simulink model "B4_quadcopter_model_discrete"  (R2021b)
settings: Solver=VariableStepAuto  StartTime=0.0  StopTime=10  FixedStep=0.002  RelTol=1e-3
values from neighbouring files (symbols this model uses):
  coef_sim_1 = tf_des_d.Denominator{1}(2)    [A11_setup_script_pprz.m]    (also in A1_setup_script.m; A6_slow_actuator.m)
  coef_sim_2 = tf_des_d.Numerator{1}(2)    [A11_setup_script_pprz.m]    (also in A1_setup_script.m; A6_slow_actuator.m)
  doublet_mag = - 0.15    (= -0.15)    [A11_setup_script_pprz.m]    (also in A1_setup_script.m)
  doublet_time = 6    [A11_setup_script_pprz.m]    (also in A1_setup_script.m)
  f_8 = 1    [A11_setup_script_pprz.m]    (also in A1_setup_script.m)
  FILT_CUTOFF = 2*pi*5    (= 31.4159265359)    [A11_setup_script_pprz.m]    (also in A1_setup_script.m)
  FILTER = 1    [A11_setup_script_pprz.m]    (also in A1_setup_script.m)
  G1 = inv(I)*G1_r    [A10_simple_plant.m]    (also in A11_setup_script_pprz.m = G1/scale; A1_setup_script.m = [G1;G1_T])
  G1_simple = inv(I)*G1_r_simple    [A1_setup_script.m]
  G2 = G2/scale    [A11_setup_script_pprz.m]    (also in A1_setup_script.m = (1/sampling_time)*inv(I)*(G2_r))
  h_plate = 0.3    [A11_setup_script_pprz.m]    (also in A1_setup_script.m = 0.16)
  I = eye(3,3)    [A10_simple_plant.m]    (also in A11_setup_script_pprz.m; A1_setup_script.m; A2_B_matrix_generation_symbolic.m = [Ixx 0 0; A3_B_matrix_generation_symbolic_cascaded.m = [Ixx 0 0)
  Iyy = 0.0008    [A11_setup_script_pprz.m]    (also in A1_setup_script.m = 0.0015)
  Izz = 0.000498    [A11_setup_script_pprz.m]    (also in A1_setup_script.m = 0.00015)
  K = 7    [A11_setup_script_pprz.m]    (also in A1_setup_script.m = 10)
  K_act = 50    [A10_simple_plant.m]    (also in A11_setup_script_pprz.m = 20; A1_setup_script.m = 20)
  K_act_outer = diag([K K K_act])    [A1_setup_script.m]
  K_d = 15    [A11_setup_script_pprz.m]    (also in A1_setup_script.m = 25)
  K_dd = K_act    (= 20)    [A11_setup_script_pprz.m]    (also in A1_setup_script.m)
  K_dyn = K    (= 10)    [A1_setup_script.m]
  K_ec = 50    [A11_setup_script_pprz.m]    (also in A1_setup_script.m = 251)
  K_ec_d = 13    [A11_setup_script_pprz.m]    (also in A1_setup_script.m = 25)
  K_ec_d_u = 1.5    [A11_setup_script_pprz.m]    (also in A1_setup_script.m = 5)
  K_ec_d_v = 1.5    [A11_setup_script_pprz.m]    (also in A1_setup_script.m = 5)
  K_ec_d_w = 1.5    [A11_setup_script_pprz.m]    (also in A1_setup_script.m = 5)
  K_ec_dd = 9    [A11_setup_script_pprz.m]    (also in A1_setup_script.m = 45)
  K_ec_i = 0    [A11_setup_script_pprz.m]    (also in A1_setup_script.m = 380)
  K_ec_u = 1.5    [A11_setup_script_pprz.m]    (also in A1_setup_script.m = 5)
  K_ec_v = 1.5    [A11_setup_script_pprz.m]    (also in A1_setup_script.m = 5)
  K_ec_w = 1.5    [A11_setup_script_pprz.m]    (also in A1_setup_script.m = 5)
  K_t = 0.0005    [A10_simple_plant.m]    (also in A11_setup_script_pprz.m = 6.557e-08; A1_setup_script.m = 6.557e-08)
  K_u = 1.0    (= 1)    [A11_setup_script_pprz.m]    (also in A1_setup_script.m = 1.5)
  K_u_d = 2.5    [A11_setup_script_pprz.m]    (also in A1_setup_script.m = 7)
  K_u_dd = K    (= 10)    [A1_setup_script.m]
  K_v = 1.0    (= 1)    [A11_setup_script_pprz.m]    (also in A1_setup_script.m = 1.5)
  K_v_d = 2.5    [A11_setup_script_pprz.m]    (also in A1_setup_script.m = 7)
  K_v_dd = K    (= 10)    [A1_setup_script.m]
  K_w = 1.0    (= 1)    [A11_setup_script_pprz.m]    (also in A1_setup_script.m = 4.5)
  K_w_d = 2.5    [A11_setup_script_pprz.m]    (also in A1_setup_script.m = 7)
  K_w_dd = K    (= 10)    [A1_setup_script.m]
  l_plate = 0.1    [A11_setup_script_pprz.m]    (also in A1_setup_script.m = 0.11)
  m = 0.4    [A10_simple_plant.m]    (also in A11_setup_script_pprz.m; A1_setup_script.m)
  NOISE = 0    [A11_setup_script_pprz.m]    (also in A1_setup_script.m)
  NOISE_ACC = 0.00005    (= 5e-05)    [A11_setup_script_pprz.m]    (also in A1_setup_script.m)
  NOISE_GYRO = 0.00005    (= 5e-05)    [A11_setup_script_pprz.m]    (also in A1_setup_script.m)
  NOISE_RPM = 200    [A11_setup_script_pprz.m]    (also in A1_setup_script.m)
  omega_act = 50    [A6_slow_actuator.m]
  omega_des = 20.00    (= 20)    [A11_setup_script_pprz.m]    (also in A1_setup_script.m; A6_slow_actuator.m = 49)
  sampling_time = 1/frequency    (= 0.002)    [A11_setup_script_pprz.m]    (also in A12_sim_multi_run.m; A1_setup_script.m; A6_slow_actuator.m)
  scale_8 = 1.6    [A11_setup_script_pprz.m]    (also in A1_setup_script.m)
  start_8 = 2    [A11_setup_script_pprz.m]    (also in A1_setup_script.m)
  start_time = 2    [A11_setup_script_pprz.m]    (also in A1_setup_script.m = 1)
  t_8 = 10    [A11_setup_script_pprz.m]    (also in A1_setup_script.m)
  w_plate = 0.3    [A11_setup_script_pprz.m]    (also in A1_setup_script.m = 0.36)
undefined symbols (not defined in the file or in its folder): DiscIntNeverNeededParam, K_ec_d_p, K_ec_d_q, K_ec_d_r, K_ec_dd_p, K_ec_dd_q, K_ec_dd_r, K_ec_i_u, K_ec_i_v, K_ec_i_w, K_ec_p, K_ec_q, K_ec_r, K_p, K_p_d, K_p_dd, K_q, K_q_d, K_q_dd, K_r, K_r_d, K_r_dd
libraries: simulink x44, cstblocks x37, dspinverses x26, dspmathops x9, dspstat3 x9, aerolibutil x9, sharedutil x3, aerolibanim x1
(part 12 of 13)

== matlab function B4_quadcopter_model_discrete/Discrete Model/Discrete INDI Controller Cascaded w// Actuator Compensation/8-shape trajectory/MATLAB Function ==
  data: x output; t input; y output; f input; scale input; psi output; sampling_time input; total_time input; start_time input
function [x,y,psi] = inf_trajectory(t,f,scale,sampling_time,total_time,start_time)

t_norm = t/total_time;

x = 2*scale*sin(2*pi*f*t_norm);
y = scale*sin(2*pi*f*t_norm*2);

x_n = 2*scale*sin(2*pi*f*(t_norm+sampling_time));
y_n = scale*sin(2*pi*f*(t_norm+sampling_time)*2);

dx = x_n - x;
dy = y_n - y;

psi = atan2(dy,dx);

== matlab function B4_quadcopter_model_discrete/Discrete Model - Complementary Filtering/Discrete INDI Controller Cascaded w// Actuator Compensation/8-shape trajectory/MATLAB Function ==
  data: x output; t input; y output; f input; scale input; psi output; sampling_time input; total_time input; start_time input
function [x,y,psi] = inf_trajectory(t,f,scale,sampling_time,total_time,start_time)

t_norm = t/total_time;

x = 2*scale*sin(2*pi*f*t_norm);
y = scale*sin(2*pi*f*t_norm*2);

x_n = 2*scale*sin(2*pi*f*(t_norm+sampling_time));
y_n = scale*sin(2*pi*f*(t_norm+sampling_time)*2);

dx = x_n - x;
dy = y_n - y;

psi = atan2(dy,dx);

== matlab function B4_quadcopter_model_discrete/Discrete Model - Complementary Filtering/Discrete INDI Controller Cascaded w// Actuator Compensation/ERROR CONTROLLER ATTITUDE/MATLAB Function1 ==
  data: pis_e input; psie_w output
function psie_w = wrapper(pis_e)

if pis_e > pi
    psie_w = pis_e - 2*pi;
elseif pis_e <= -pi
    psie_w = pis_e + 2*pi;
else
    psie_w = pis_e;
end

== matlab function B4_quadcopter_model_discrete/Discrete Model/Discrete INDI Controller Cascaded w// Actuator Compensation Double/Pitch Jerk Compensation1/MATLAB Function ==
  data: Ax input; dtheta input; Vx input; theta input; Jx_comp output; w_plate input; h_plate input; m input
function Jx_comp = jerk_compensator(Ax,dtheta,Vx,theta,w_plate,h_plate,m)

S_plate = w_plate * h_plate;
rho = 1.225;
Vx_sign = sign(Vx);

Jx_comp = - (297*S_plate*Vx^2*Vx_sign*dtheta*rho)/(1000*m*pi) - (Ax*S_plate*Vx*Vx_sign*rho*((297*theta)/(500*pi) + 997/1000))/m;

== matlab function B4_quadcopter_model_discrete/Discrete Model/Discrete INDI Controller Cascaded w// Actuator Compensation Double/8-shape trajectory/MATLAB Function ==
  data: x output; t input; y output; f input; scale input; psi output; sampling_time input; total_time input; start_time input
function [x,y,psi] = inf_trajectory(t,f,scale,sampling_time,total_time,start_time)

t_norm = t/total_time;

x = 2*scale*sin(2*pi*f*t_norm);
y = scale*sin(2*pi*f*t_norm*2);

x_n = 2*scale*sin(2*pi*f*(t_norm+sampling_time));
y_n = scale*sin(2*pi*f*(t_norm+sampling_time)*2);

dx = x_n - x;
dy = y_n - y;

psi = atan2(dy,dx);

if psi > 2
    psi = psi - 2*pi;
end

== matlab function B4_quadcopter_model_discrete/Discrete Model/Discrete INDI Controller Cascaded w// Actuator Compensation Double/Drag Plate Aerodynamics/drag plate My ==
  data: w_plate input; h_plate input; l_plate input; theta input; Vx input; My_dp output; Fx_earth output; Fz_earth output; Cl output; Cd output
function [My_dp, Fx_earth, Fz_earth, Cl, Cd]= drag_plate_My(w_plate,h_plate,l_plate,theta,Vx)

% define constants
rho = 1.225;
S_plate = w_plate*h_plate;

% Drag Coefficient
Cd = 0.0033*(90+rad2deg(theta))+0.7;

% Lift Coefficient
Cl = -0.0228*(90+rad2deg(theta))+2.01;

% get drag and lift
D_plate = 0.5*rho*Vx^2*S_plate*Cd;
L_plate = 0.5*rho*Vx^2*S_plate*Cl;
R_plate = sqrt(D_plate^2 + L_plate^2);

% get the moment caused by the drag
My_dp = l_plate*R_plate;

% get the forces caused by the drag
Fx_earth = -D_plate*sign(Vx);
Fz_earth = -L_plate;

== matlab function B4_quadcopter_model_discrete/Discrete Model/Discrete INDI Controller Cascaded w// Actuator Compensation/body rates to euler rates/pqr_to_euler_rates ==
  data: Phi input; T output; Theta input
function T = pqr_to_euler_rates(Phi,Theta)
T = [1 (sin(Phi)*sin(Theta))/cos(Theta) (cos(Phi)*sin(Theta))/cos(Theta);
0 cos(Phi) -sin(Phi);
0 sin(Phi)/cos(Theta) cos(Phi)/cos(Theta)];

== matlab function B4_quadcopter_model_discrete/Discrete Model/Discrete INDI Controller Cascaded w// Actuator Compensation Double/G1+G2 ==
  data: G1 input; B_inner output; G2 input; omega input; K_act input
function B_inner = B_inner(G1,G2,omega,K_act)

% add additional row to G2 for equal size
G2_T = [0 0 0 0];
G2 = vertcat(G2,G2_T);

B_inner = K_act*(G1 .* omega' + G2);

== matlab function B4_quadcopter_model_discrete/Discrete Model/Discrete INDI Controller Cascaded w// Actuator Compensation Double/G2_comp ==
  data: G2 input; K_act input; domega input; G2_comp output
function G2_comp = G2_comp(G2,K_act,domega)

G2_comp = K_act * G2(3,:) * domega;

== matlab function B4_quadcopter_model_discrete/Discrete Model/Discrete INDI Controller Cascaded w// Actuator Compensation Double/MATLAB Function1 ==
  data: T input; B_outer output; Phi input; Theta input; Psi input; m input; K_act_outer input
function B_outer = control_allocation_simple_outer(T,Phi,Theta,Psi,m,K_act_outer)

B_outer = zeros(3,3);

B_outer(1,1) = (T*cos(Phi)*cos(Psi)*cos(Theta))/m;
B_outer(2,1) = (T*cos(Phi)*cos(Theta)*sin(Psi))/m;
B_outer(3,1) = -(T*cos(Phi)*sin(Theta))/m;

B_outer(1,2) = (T*(cos(Phi)*sin(Psi) - cos(Psi)*sin(Phi)*sin(Theta)))/m;
B_outer(2,2) = -(T*(cos(Phi)*cos(Psi) + sin(Phi)*sin(Psi)*sin(Theta)))/m;
B_outer(3,2) = -(T*cos(Theta)*sin(Phi))/m;

B_outer(1,3) = (sin(Phi)*sin(Psi) + cos(Phi)*cos(Psi)*sin(Theta))/m;
B_outer(2,3) = -(cos(Psi)*sin(Phi) - cos(Phi)*sin(Psi)*sin(Theta))/m;
B_outer(3,3) = (cos(Phi)*cos(Theta))/m;

% compensate for actuator dynamics
B_outer = K_act_outer * B_outer;

end

== matlab function B4_quadcopter_model_discrete/Discrete Model/Discrete INDI Controller Cascaded w// Actuator Compensation Double/Pitch Jerk Compensation/MATLAB Function ==
  data: dx input; dy input; dz input; Phi input; Theta input; Psi input; ddx input; ddy input; ddz input; dPhi input; dTheta input; dPsi input; qdd_comp output; w_plate input; h_plate input; l_plate input; Iyy input
function qdd_comp = pitch_compensator(dx,dy,dz,Phi,Theta,Psi,ddx,ddy,ddz,dPhi,dTheta,dPsi,w_plate,h_plate,l_plate,Iyy)

% define constants
rho = 1.225;
S_plate = w_plate*h_plate;
Cd = 1.2;
Cl = 0.2;

% Q term
Q = (l_plate*rho*S_plate)/(Iyy*2);

% derivative vector
der_vect = [ddx ddy ddz dPhi dTheta dPsi];

% State terms
Fs_theta_dx = -Q*(Cd*cos(Theta) - Cl*sin(Theta))*(2*(sin(Phi)*sin(Psi) + cos(Phi)*cos(Psi)*sin(Theta))*(dx*(sin(Phi)*sin(Psi) + cos(Phi)*cos(Psi)*sin(Theta)) - dy*(cos(Psi)*sin(Phi) - cos(Phi)*sin(Psi)*sin(Theta)) + dz*cos(Phi)*cos(Theta)) + 2*cos(Psi)*cos(Theta)*(dx*cos(Psi)*cos(Theta) - dz*sin(Theta) + dy*cos(Theta)*sin(Psi)));
Fs_theta_dy = Q*(Cd*cos(Theta) - Cl*sin(Theta))*(2*(cos(Psi)*sin(Phi) - cos(Phi)*sin(Psi)*sin(Theta))*(dx*(sin(Phi)*sin(Psi) + cos(Phi)*cos(Psi)*sin(Theta)) - dy*(cos(Psi)*sin(Phi) - cos(Phi)*sin(Psi)*sin(Theta)) + dz*cos(Phi)*cos(Theta)) - 2*cos(Theta)*sin(Psi)*(dx*cos(Psi)*cos(Theta) - dz*sin(Theta) + dy*cos(Theta)*sin(Psi)));
Fs_theta_dz = Q*(Cd*cos(Theta) - Cl*sin(Theta))*(2*sin(Theta)*(dx*cos(Psi)*cos(Theta) - dz*sin(Theta) + dy*cos(Theta)*sin(Psi)) - 2*cos(Phi)*cos(Theta)*(dx*(sin(Phi)*sin(Psi) + cos(Phi)*cos(Psi)*sin(Theta)) - dy*(cos(Psi)*sin(Phi) - cos(Phi)*sin(Psi)*sin(Theta)) + dz*cos(Phi)*cos(Theta)));
Fs_theta_phi = 2*Q*(Cd*cos(Theta) - Cl*sin(Theta))*(dx*(sin(Phi)*sin(Psi) + cos(Phi)*cos(Psi)*sin(Theta)) - dy*(cos(Psi)*sin(Phi) - cos(Phi)*sin(Psi)*sin(Theta)) + dz*cos(Phi)*cos(Theta))*(dy*(cos(Phi)*cos(Psi) + sin(Phi)*sin(Psi)*sin(Theta)) - dx*(cos(Phi)*sin(Psi) - cos(Psi)*sin(Phi)*sin(Theta)) + dz*cos(Theta)*sin(Phi));
Fs_theta_theta = Q*(Cl*cos(Theta) + Cd*sin(Theta))*((dx*(sin(Phi)*sin(Psi) + cos(Phi)*cos(Psi)*sin(Theta)) - dy*(cos(Psi)*sin(Phi) - cos(Phi)*sin(Psi)*sin(Theta)) + dz*cos(Phi)*cos(Theta))^2 + (dx*cos(Psi)*cos(Theta) - dz*sin(Theta) + dy*cos(Theta)*sin(Psi))^2) + Q*(2*(dx*cos(Psi)*cos(Theta) - dz*sin(Theta) + dy*cos(Theta)*sin(Psi))*(dz*cos(Theta) + dx*cos(Psi)*sin(Theta) + dy*sin(Psi)*sin(Theta)) - 2*(dx*cos(Phi)*cos(Psi)*cos(Theta) - dz*cos(Phi)*sin(Theta) + dy*cos(Phi)*cos(Theta)*sin(Psi))*(dx*(sin(Phi)*sin(Psi) + cos(Phi)*cos(Psi)*sin(Theta)) - dy*(cos(Psi)*sin(Phi) - cos(Phi)*sin(Psi)*sin(Theta)) + dz*cos(Phi)*cos(Theta)))*(Cd*cos(Theta) - Cl*sin(Theta));
Fs_theta_psi = -Q*(Cd*cos(Theta) - Cl*sin(Theta))*(2*(dy*cos(Psi)*cos(Theta) - dx*cos(Theta)*sin(Psi))*(dx*cos(Psi)*cos(Theta) - dz*sin(Theta) + dy*cos(Theta)*sin(Psi)) + 2*(dx*(cos(Psi)*sin(Phi) - cos(Phi)*sin(Psi)*sin(Theta)) + dy*(sin(Phi)*sin(Psi) + cos(Phi)*cos(Psi)*sin(Theta)))*(dx*(sin(Phi)*sin(Psi) + cos(Phi)*cos(Psi)*sin(Theta)) - dy*(cos(Psi)*sin(Phi) - cos(Phi)*sin(Psi)*sin(Theta)) + dz*cos(Phi)*cos(Theta)));

Fs_theta_der = [Fs_theta_dx Fs_theta_dy Fs_theta_dz Fs_theta_phi Fs_theta_theta Fs_theta_psi];

% compensation term
qdd_comp = Fs_theta_der * der_vect';

== matlab function B4_quadcopter_model_discrete/Discrete Model/Discrete INDI Controller Cascaded w// Actuator Compensation Double/Pitch Jerk Compensation CopyPaste/Aero Package Easy/drag plate My ==
  data: w_plate input; h_plate input; l_plate input; theta input; u input; w input; My_dp output; Fx_earth output; Fz_earth output; Cl output; Cd output
function [My_dp, Fx_earth, Fz_earth, Cl, Cd]= drag_plate_My(w_plate,h_plate,l_plate,theta,u,w)

% define constants
rho = 1.225;
S_plate = w_plate*h_plate;

% Velocity vector
V = sqrt(u^2+w^2);

% % Drag Coefficient
% Cd = 0.0033*(90+rad2deg(theta))+0.7;
% 
% % Lift Coefficient
% Cl = -0.0228*(90+rad2deg(theta))+2.01;

Cd = 1.2;
Cl = 0.2;

% get drag and lift
D_plate = 0.5*rho*V^2*S_plate*Cd*sign(u);
L_plate = 0.5*rho*V^2*S_plate*Cl;

% get forces in body frame
Fx_body = - D_plate * cos(theta) + L_plate * sin(theta);
Fz_body = - D_plate * sin(theta) - L_plate * cos(theta);

% get the moment caused by the drag
My_dp = l_plate*Fx_body;

% get the forces caused by the drag
Fx_earth = - D_plate;
Fz_earth = L_plate;

== matlab function B4_quadcopter_model_discrete/Tester Block/Wrapping Test/MATLAB Function ==
  data: x output; t input; y output; f input; scale input; psi output; sampling_time input; total_time input; start_time input
function [x,y,psi] = inf_trajectory(t,f,scale,sampling_time,total_time,start_time)

t_norm = t/total_time;

x = 2*scale*sin(2*pi*f*t_norm);
y = scale*sin(2*pi*f*t_norm*2);

x_n = 2*scale*sin(2*pi*f*(t_norm+sampling_time));
y_n = scale*sin(2*pi*f*(t_norm+sampling_time)*2);

dx = x_n - x;
dy = y_n - y;

psi = atan2(dy,dx);

== matlab function B4_quadcopter_model_discrete/Discrete Model/Discrete INDI Controller Cascaded/G1+G2 ==
  data: G1 input; B_inner output; G2 input; omega input
function B_inner = B_inner(G1,G2,omega)

% add additional row to G2 for equal size
G2_T = [0 0 0 0];
G2 = vertcat(G2,G2_T);

B_inner = (G1 .* omega' + G2);

== matlab function B4_quadcopter_model_discrete/Tester Block/Wrapping Test/MATLAB Function1 ==
  data: pis_e input; psie_w output
function psie_w = wrapper(pis_e)

if pis_e > pi
    psie_w = pis_e - 2*pi;
elseif pis_e <= -pi
    psie_w = pis_e + 2*pi;
else
    psie_w = pis_e;
end

== matlab function B4_quadcopter_model_discrete/Tester Block/Wrapping Test/MATLAB Function2 ==
  data: psi_e_w input; psi_e output
function psi_e = unwrap(psi_e_w)

if psi_e_w > pi
    psi_e = psi_e_w - 2*pi;
elseif psi_e_w <= -pi
    psi_e = psi_e_w + 2*pi;
else
    psi_e = psi_e_w;
end

== matlab function B4_quadcopter_model_discrete/Discrete Model/Discrete INDI Controller Cascaded w// Actuator Compensation/INTERNAL REFERENCE MODEL ATTITUDE/MATLAB Function1 ==
  data: pis_e input; psie_w output
function psie_w = wrapper(pis_e)

if pis_e > pi
    psie_w = pis_e - 2*pi;
elseif pis_e <= -pi
    psie_w = pis_e + 2*pi;
else
    psie_w = pis_e;
end

== matlab function B4_quadcopter_model_discrete/Discrete Model/Plant and State Estimation/euler_rates_to_pqr ==
  data: Phi input; R output; Theta input
function R = euler_rates_to_pqr(Phi,Theta)
R = [1 0 -sin(Theta);
0 cos(Phi) cos(Theta)*sin(Phi);
0 -sin(Phi) cos(Phi)*cos(Theta)];

== matlab function B4_quadcopter_model_discrete/Discrete Model/Plant and State Estimation/pqr_to_euler_rates ==
  data: Phi input; T output; Theta input
function T = pqr_to_euler_rates(Phi,Theta)
T = [1 (sin(Phi)*sin(Theta))/cos(Theta) (cos(Phi)*sin(Theta))/cos(Theta);
0 cos(Phi) -sin(Phi);
0 sin(Phi)/cos(Theta) cos(Phi)/cos(Theta)];

== matlab function B4_quadcopter_model_discrete/Discrete Model/Discrete INDI Controller Cascaded/MATLAB Function1 ==
  data: T input; B_outer output; Phi input; Theta input; Psi input; m input
function B_outer = control_allocation_simple_outer(T,Phi,Theta,Psi,m)

B_outer = zeros(3,3);

% matrix obtained in ZXY rotation
% output order u = [phi theta thrust]
B_outer(1,1) = (T*cos(Phi)*cos(Psi)*cos(Theta))/m;
B_outer(2,1) = (T*cos(Phi)*cos(Theta)*sin(Psi))/m;
B_outer(3,1) = -(T*cos(Phi)*sin(Theta))/m;

B_outer(1,2) = (T*(cos(Phi)*sin(Psi) - cos(Psi)*sin(Phi)*sin(Theta)))/m;
B_outer(2,2) = -(T*(cos(Phi)*cos(Psi) + sin(Phi)*sin(Psi)*sin(Theta)))/m;
B_outer(3,2) = -(T*cos(Theta)*sin(Phi))/m;

B_outer(1,3) = (sin(Phi)*sin(Psi) + cos(Phi)*cos(Psi)*sin(Theta))/m;
B_outer(2,3) = -(cos(Psi)*sin(Phi) - cos(Phi)*sin(Psi)*sin(Theta))/m;
B_outer(3,3) = (cos(Phi)*cos(Theta))/m;

end

== matlab function B4_quadcopter_model_discrete/Discrete Model/Plant and State Estimation/wrapper ==
  data: pis_e input; psie_w output
function psie_w = wrapper(pis_e)

if pis_e > pi
    psie_w = pis_e - 2*pi;
elseif pis_e <= -pi
    psie_w = pis_e + 2*pi;
else
    psie_w = pis_e;
end

== matlab function B4_quadcopter_model_discrete/Discrete Model/Plant and State Estimation/wrapper1 ==
  data: pis_e input; psie_w output
function psie_w = wrapper(pis_e)

if pis_e > pi
    psie_w = pis_e - 2*pi;
elseif pis_e <= -pi
    psie_w = pis_e + 2*pi;
else
    psie_w = pis_e;
end

== matlab function B4_quadcopter_model_discrete/Discrete Model/Discrete INDI Controller Cascaded w// Actuator Compensation/ERROR CONTROLLER ATTITUDE/MATLAB Function1 ==
  data: pis_e input; psie_w output
function psie_w = wrapper(pis_e)

if pis_e > pi
    psie_w = pis_e - 2*pi;
elseif pis_e <= -pi
    psie_w = pis_e + 2*pi;
else
    psie_w = pis_e;
end

== matlab function B4_quadcopter_model_discrete/Discrete Model/Discrete INDI Controller Cascaded/INTERNAL REFERENCE MODEL ATTITUDE/MATLAB Function1 ==
  data: pis_e input; psie_w output
function psie_w = wrapper(pis_e)

if pis_e > pi
    psie_w = pis_e - 2*pi;
elseif pis_e <= -pi
    psie_w = pis_e + 2*pi;
else
    psie_w = pis_e;
end

== matlab function B4_quadcopter_model_discrete/Discrete Model/Discrete INDI Controller Cascaded/ERROR CONTROLLER ATTITUDE/MATLAB Function1 ==
  data: pis_e input; psie_w output
function psie_w = wrapper(pis_e)

if pis_e > pi
    psie_w = pis_e - 2*pi;
elseif pis_e <= -pi
    psie_w = pis_e + 2*pi;
else
    psie_w = pis_e;
end

== matlab function B4_quadcopter_model_discrete/Discrete Model/Force and Moment Calculation/Moments due to thrust ==
  data: omega input; omega_dot input; M_t output; G1 input; G2 input; sampling_time input; I input
function M_t = M_t(omega, omega_dot, G1, G2, sampling_time, I)

M_t = I * (0.5 * G1(1:3,:) * omega.^2 + sampling_time * G2 * omega_dot);

== matlab function B4_quadcopter_model_discrete/Discrete Model/Plant and State Estimation/Plant Dynamics Continuous/wrapper ==
  data: pis_e input; psie_w output
function psie_w = wrapper(pis_e)

if pis_e > pi
    psie_w = pis_e - 2*pi;
elseif pis_e <= -pi
    psie_w = pis_e + 2*pi;
else
    psie_w = pis_e;
end

== matlab function B4_quadcopter_model_discrete/Discrete Model - Complementary Filtering/Discrete INDI Controller Cascaded w// Actuator Compensation/G1+G2 ==
  data: G1 input; B_inner output; G2 input; omega input; K_act input
function B_inner = B_inner(G1,G2,omega,K_act)

% add additional row to G2 for equal size
G2_T = [0 0 0 0];
G2 = vertcat(G2,G2_T);

B_inner = K_act*(G1 .* omega' + G2);

== matlab function B4_quadcopter_model_discrete/Discrete Model - Complementary Filtering/Discrete INDI Controller Cascaded w// Actuator Compensation/G2_comp ==
  data: G2 input; K_act input; domega input; G2_comp output
function G2_comp = G2_comp(G2,K_act,domega)

G2_comp = K_act * G2(3,:) * domega;

== matlab function B4_quadcopter_model_discrete/Discrete Model - Complementary Filtering/Discrete INDI Controller Cascaded w// Actuator Compensation/INTERNAL REFERENCE MODEL ATTITUDE/MATLAB Function1 ==
  data: pis_e input; psie_w output
function psie_w = wrapper(pis_e)

if pis_e > pi
    psie_w = pis_e - 2*pi;
elseif pis_e <= -pi
    psie_w = pis_e + 2*pi;
else
    psie_w = pis_e;
end

== matlab function B4_quadcopter_model_discrete/Discrete Model - Complementary Filtering/Discrete INDI Controller Cascaded w// Actuator Compensation/MATLAB Function1 ==
  data: T input; B_outer output; Phi input; Theta input; Psi input; m input
function B_outer = control_allocation_simple_outer(T,Phi,Theta,Psi,m)

B_outer = zeros(3,3);

% matrix obtained in ZXY rotation
% output order u = [phi theta thrust]
B_outer(1,1) = (T*cos(Phi)*cos(Psi)*cos(Theta))/m;
B_outer(2,1) = (T*cos(Phi)*cos(Theta)*sin(Psi))/m;
B_outer(3,1) = -(T*cos(Phi)*sin(Theta))/m;

B_outer(1,2) = (T*(cos(Phi)*sin(Psi) - cos(Psi)*sin(Phi)*sin(Theta)))/m;
B_outer(2,2) = -(T*(cos(Phi)*cos(Psi) + sin(Phi)*sin(Psi)*sin(Theta)))/m;
B_outer(3,2) = -(T*cos(Theta)*sin(Phi))/m;

B_outer(1,3) = (sin(Phi)*sin(Psi) + cos(Phi)*cos(Psi)*sin(Theta))/m;
B_outer(2,3) = -(cos(Psi)*sin(Phi) - cos(Phi)*sin(Psi)*sin(Theta))/m;
B_outer(3,3) = (cos(Phi)*cos(Theta))/m;

end

== matlab function B4_quadcopter_model_discrete/Discrete Model - Complementary Filtering/Plant and State Estimation/Angular Velocity Model/Drag Plate Aerodynamics/drag plate My ==
  data: w_plate input; h_plate input; l_plate input; theta input; Vx input; Mz_dp output; Fx_earth output; Fy_earth output; Fz_earth output; Vy input; heading input; q input; D_plate_vel output; D_plate_rot output
function [Mz_dp, Fx_earth, Fy_earth, Fz_earth, D_plate_vel, D_plate_rot] = drag_plate_My(w_plate,h_plate,l_plate,theta,Vx,Vy,heading,q)

% define constants
rho = 1.225;
S_plate = w_plate*h_plate;

% Drag Coefficient
Cd = 0.0033*(90+rad2deg(theta))+0.7;

% Lift Coefficient
Cl = -0.0228*(90+rad2deg(theta))+2.01;

% Resultant
Vr = sqrt(Vx^2+Vy^2);

% get drag and lift
D_plate_vel = 0.5*rho*Vr^2*S_plate*Cd;
D_plate_rot = 0.5*rho*(q*l_plate)^2*S_plate*Cd;
L_plate = 0.5*rho*Vr^2*S_plate*Cl;
R_plate = sqrt(D_plate_vel^2 + L_plate^2);

% get the moment caused by the drag
% My_dp = l_plate*R_plate + l_plate*D_plate_rot;
Mz_dp = -(0.095+l_plate)*R_plate;
D_x = D_plate_vel*cos(heading);
D_y = D_plate_vel*sin(heading);

% get the forces caused by the drag
Fx_earth = -D_x;
Fy_earth = -D_y;
Fz_earth = -L_plate;

== matlab function B4_quadcopter_model_discrete/Discrete Model - Complementary Filtering/Discrete INDI Controller Cascaded w// Actuator Compensation Double/8-shape trajectory/MATLAB Function ==
  data: x output; t input; y output; f input; scale input; psi output; sampling_time input; total_time input; start_time input
function [x,y,psi] = inf_trajectory(t,f,scale,sampling_time,total_time,start_time)

t_norm = t/total_time;

x = 2*scale*sin(2*pi*f*t_norm);
y = scale*sin(2*pi*f*t_norm*2);

x_n = 2*scale*sin(2*pi*f*(t_norm+sampling_time));
y_n = scale*sin(2*pi*f*(t_norm+sampling_time)*2);

dx = x_n - x;
dy = y_n - y;

psi = atan2(dy,dx);

if psi > 2
    psi = psi - 2*pi;
end

== matlab function B4_quadcopter_model_discrete/Discrete Model - Complementary Filtering/Discrete INDI Controller Cascaded w// Actuator Compensation Double/Drag Plate Aerodynamics/drag plate My ==
  data: w_plate input; h_plate input; l_plate input; theta input; Vx input; My_dp output; Fx_earth output; Fz_earth output; Cl output; Cd output
function [My_dp, Fx_earth, Fz_earth, Cl, Cd]= drag_plate_My(w_plate,h_plate,l_plate,theta,Vx)

% define constants
rho = 1.225;
S_plate = w_plate*h_plate;

% Drag Coefficient
Cd = 0.0033*(90+rad2deg(theta))+0.7;

% Lift Coefficient
Cl = -0.0228*(90+rad2deg(theta))+2.01;

% get drag and lift
D_plate = 0.5*rho*Vx^2*S_plate*Cd;
L_plate = 0.5*rho*Vx^2*S_plate*Cl;
R_plate = sqrt(D_plate^2 + L_plate^2);

% get the moment caused by the drag
My_dp = l_plate*R_plate;

% get the forces caused by the drag
Fx_earth = -D_plate*sign(Vx);
Fz_earth = -L_plate;

== matlab function B4_quadcopter_model_discrete/Discrete Model - Complementary Filtering/Discrete INDI Controller Cascaded w// Actuator Compensation Double/G1+G2 ==
  data: G1 input; B_inner output; G2 input; omega input; K_act input
function B_inner = B_inner(G1,G2,omega,K_act)

% add additional row to G2 for equal size
G2_T = [0 0 0 0];
G2 = vertcat(G2,G2_T);

B_inner = K_act*(G1 .* omega' + G2);

== matlab function B4_quadcopter_model_discrete/Discrete Model - Complementary Filtering/Discrete INDI Controller Cascaded w// Actuator Compensation Double/G2_comp ==
  data: G2 input; K_act input; domega input; G2_comp output
function G2_comp = G2_comp(G2,K_act,domega)

G2_comp = K_act * G2(3,:) * domega;

== matlab function B4_quadcopter_model_discrete/Discrete Model - Complementary Filtering/Discrete INDI Controller Cascaded w// Actuator Compensation Double/MATLAB Function1 ==
  data: T input; B_outer output; Phi input; Theta input; Psi input; m input; K_act_outer input
function B_outer = control_allocation_simple_outer(T,Phi,Theta,Psi,m,K_act_outer)

B_outer = zeros(3,3);

B_outer(1,1) = (T*cos(Phi)*cos(Psi)*cos(Theta))/m;
B_outer(2,1) = (T*cos(Phi)*cos(Theta)*sin(Psi))/m;
B_outer(3,1) = -(T*cos(Phi)*sin(Theta))/m;

B_outer(1,2) = (T*(cos(Phi)*sin(Psi) - cos(Psi)*sin(Phi)*sin(Theta)))/m;
B_outer(2,2) = -(T*(cos(Phi)*cos(Psi) + sin(Phi)*sin(Psi)*sin(Theta)))/m;
B_outer(3,2) = -(T*cos(Theta)*sin(Phi))/m;

B_outer(1,3) = (sin(Phi)*sin(Psi) + cos(Phi)*cos(Psi)*sin(Theta))/m;
B_outer(2,3) = -(cos(Psi)*sin(Phi) - cos(Phi)*sin(Psi)*sin(Theta))/m;
B_outer(3,3) = (cos(Phi)*cos(Theta))/m;

% compensate for actuator dynamics
B_outer = K_act_outer * B_outer;

end

== matlab function B4_quadcopter_model_discrete/Discrete Model - Complementary Filtering/Discrete INDI Controller Cascaded/8-shape trajectory/MATLAB Function ==
  data: x output; t input; y output; f input; scale input; psi output; sampling_time input; total_time input; start_time input
function [x,y,psi] = inf_trajectory(t,f,scale,sampling_time,total_time,start_time)

t_norm = t/total_time;

x = 2*scale*sin(2*pi*f*t_norm);
y = scale*sin(2*pi*f*t_norm*2);

x_n = 2*scale*sin(2*pi*f*(t_norm+sampling_time));
y_n = scale*sin(2*pi*f*(t_norm+sampling_time)*2);

dx = x_n - x;
dy = y_n - y;

psi = atan2(dy,dx);

== matlab function B4_quadcopter_model_discrete/Discrete Model - Complementary Filtering/Discrete INDI Controller Cascaded w// Actuator Compensation Double/Pitch Jerk Compensation/MATLAB Function ==
  data: dx input; dy input; dz input; Phi input; Theta input; Psi input; ddx input; ddy input; ddz input; dPhi input; dTheta input; dPsi input; qdd_comp output; w_plate input; h_plate input; l_plate input; Iyy input
function qdd_comp = pitch_compensator(dx,dy,dz,Phi,Theta,Psi,ddx,ddy,ddz,dPhi,dTheta,dPsi,w_plate,h_plate,l_plate,Iyy)

% define constants
rho = 1.225;
S_plate = w_plate*h_plate;
Cd = 1.2;
Cl = 0.2;

% Q term
Q = (l_plate*rho*S_plate)/(Iyy*2);

% derivative vector
der_vect = [ddx ddy ddz dPhi dTheta dPsi];

% State terms
Fs_theta_dx = -Q*(Cd*cos(Theta) - Cl*sin(Theta))*(2*(sin(Phi)*sin(Psi) + cos(Phi)*cos(Psi)*sin(Theta))*(dx*(sin(Phi)*sin(Psi) + cos(Phi)*cos(Psi)*sin(Theta)) - dy*(cos(Psi)*sin(Phi) - cos(Phi)*sin(Psi)*sin(Theta)) + dz*cos(Phi)*cos(Theta)) + 2*cos(Psi)*cos(Theta)*(dx*cos(Psi)*cos(Theta) - dz*sin(Theta) + dy*cos(Theta)*sin(Psi)));
Fs_theta_dy = Q*(Cd*cos(Theta) - Cl*sin(Theta))*(2*(cos(Psi)*sin(Phi) - cos(Phi)*sin(Psi)*sin(Theta))*(dx*(sin(Phi)*sin(Psi) + cos(Phi)*cos(Psi)*sin(Theta)) - dy*(cos(Psi)*sin(Phi) - cos(Phi)*sin(Psi)*sin(Theta)) + dz*cos(Phi)*cos(Theta)) - 2*cos(Theta)*sin(Psi)*(dx*cos(Psi)*cos(Theta) - dz*sin(Theta) + dy*cos(Theta)*sin(Psi)));
Fs_theta_dz = Q*(Cd*cos(Theta) - Cl*sin(Theta))*(2*sin(Theta)*(dx*cos(Psi)*cos(Theta) - dz*sin(Theta) + dy*cos(Theta)*sin(Psi)) - 2*cos(Phi)*cos(Theta)*(dx*(sin(Phi)*sin(Psi) + cos(Phi)*cos(Psi)*sin(Theta)) - dy*(cos(Psi)*sin(Phi) - cos(Phi)*sin(Psi)*sin(Theta)) + dz*cos(Phi)*cos(Theta)));
Fs_theta_phi = 2*Q*(Cd*cos(Theta) - Cl*sin(Theta))*(dx*(sin(Phi)*sin(Psi) + cos(Phi)*cos(Psi)*sin(Theta)) - dy*(cos(Psi)*sin(Phi) - cos(Phi)*sin(Psi)*sin(Theta)) + dz*cos(Phi)*cos(Theta))*(dy*(cos(Phi)*cos(Psi) + sin(Phi)*sin(Psi)*sin(Theta)) - dx*(cos(Phi)*sin(Psi) - cos(Psi)*sin(Phi)*sin(Theta)) + dz*cos(Theta)*sin(Phi));
Fs_theta_theta = Q*(Cl*cos(Theta) + Cd*sin(Theta))*((dx*(sin(Phi)*sin(Psi) + cos(Phi)*cos(Psi)*sin(Theta)) - dy*(cos(Psi)*sin(Phi) - cos(Phi)*sin(Psi)*sin(Theta)) + dz*cos(Phi)*cos(Theta))^2 + (dx*cos(Psi)*cos(Theta) - dz*sin(Theta) + dy*cos(Theta)*sin(Psi))^2) + Q*(2*(dx*cos(Psi)*cos(Theta) - dz*sin(Theta) + dy*cos(Theta)*sin(Psi))*(dz*cos(Theta) + dx*cos(Psi)*sin(Theta) + dy*sin(Psi)*sin(Theta)) - 2*(dx*cos(Phi)*cos(Psi)*cos(Theta) - dz*cos(Phi)*sin(Theta) + dy*cos(Phi)*cos(Theta)*sin(Psi))*(dx*(sin(Phi)*sin(Psi) + cos(Phi)*cos(Psi)*sin(Theta)) - dy*(cos(Psi)*sin(Phi) - cos(Phi)*sin(Psi)*sin(Theta)) + dz*cos(Phi)*cos(Theta)))*(Cd*cos(Theta) - Cl*sin(Theta));
Fs_theta_psi = -Q*(Cd*cos(Theta) - Cl*sin(Theta))*(2*(dy*cos(Psi)*cos(Theta) - dx*cos(Theta)*sin(Psi))*(dx*cos(Psi)*cos(Theta) - dz*sin(Theta) + dy*cos(Theta)*sin(Psi)) + 2*(dx*(cos(Psi)*sin(Phi) - cos(Phi)*sin(Psi)*sin(Theta)) + dy*(sin(Phi)*sin(Psi) + cos(Phi)*cos(Psi)*sin(Theta)))*(dx*(sin(Phi)*sin(Psi) + cos(Phi)*cos(Psi)*sin(Theta)) - dy*(cos(Psi)*sin(Phi) - cos(Phi)*sin(Psi)*sin(Theta)) + dz*cos(Phi)*cos(Theta)));

Fs_theta_der = [Fs_theta_dx Fs_theta_dy Fs_theta_dz Fs_theta_phi Fs_theta_theta Fs_theta_psi];

% compensation term
qdd_comp = Fs_theta_der * der_vect';

== matlab function B4_quadcopter_model_discrete/Discrete Model - Complementary Filtering/Discrete INDI Controller Cascaded w// Actuator Compensation Double/Pitch Jerk Compensation CopyPaste/Aero Package Easy/drag plate My ==
  data: w_plate input; h_plate input; l_plate input; theta input; u input; w input; My_dp output; Fx_earth output; Fz_earth output; Cl output; Cd output
function [My_dp, Fx_earth, Fz_earth, Cl, Cd]= drag_plate_My(w_plate,h_plate,l_plate,theta,u,w)

% define constants
rho = 1.225;
S_plate = w_plate*h_plate;

% Velocity vector
V = sqrt(u^2+w^2);

% % Drag Coefficient
% Cd = 0.0033*(90+rad2deg(theta))+0.7;
% 
% % Lift Coefficient
% Cl = -0.0228*(90+rad2deg(theta))+2.01;

Cd = 1.2;
Cl = 0.2;

% get drag and lift
D_plate = 0.5*rho*V^2*S_plate*Cd*sign(u);
L_plate = 0.5*rho*V^2*S_plate*Cl;

% get forces in body frame
Fx_body = - D_plate * cos(theta) + L_plate * sin(theta);
Fz_body = - D_plate * sin(theta) - L_plate * cos(theta);

% get the moment caused by the drag
My_dp = l_plate*Fx_body;

% get the forces caused by the drag
Fx_earth = - D_plate;
Fz_earth = L_plate;

== matlab function B4_quadcopter_model_discrete/Discrete Model - Complementary Filtering/Discrete INDI Controller Cascaded w// Actuator Compensation Double/Pitch Jerk Compensation1/MATLAB Function ==
  data: Ax input; dtheta input; Vx input; theta input; Jx_comp output; w_plate input; h_plate input; m input
function Jx_comp = jerk_compensator(Ax,dtheta,Vx,theta,w_plate,h_plate,m)

S_plate = w_plate * h_plate;
rho = 1.225;
Vx_sign = sign(Vx);

Jx_comp = - (297*S_plate*Vx^2*Vx_sign*dtheta*rho)/(1000*m*pi) - (Ax*S_plate*Vx*Vx_sign*rho*((297*theta)/(500*pi) + 997/1000))/m;

== matlab function B4_quadcopter_model_discrete/Discrete Model - Complementary Filtering/Force and Moment Calculation/Drag Plate Aerodynamics/drag plate My ==
  data: w_plate input; h_plate input; l_plate input; theta input; Vx input; Mz_dp output; Fx_earth output; Fy_earth output; Fz_earth output; Vy input; heading input; q input; D_plate_vel output; D_plate_rot output
function [Mz_dp, Fx_earth, Fy_earth, Fz_earth, D_plate_vel, D_plate_rot] = drag_plate_My(w_plate,h_plate,l_plate,theta,Vx,Vy,heading,q)

% define constants
rho = 1.225;
S_plate = w_plate*h_plate;

% Drag Coefficient
Cd = 0.0033*(90+rad2deg(theta))+0.7;

% Lift Coefficient
Cl = -0.0228*(90+rad2deg(theta))+2.01;

% Resultant
Vr = sqrt(Vx^2+Vy^2);

% get drag and lift
D_plate_vel = 0.5*rho*Vr^2*S_plate*Cd;
D_plate_rot = 0.5*rho*(q*l_plate)^2*S_plate*Cd;
L_plate = 0.5*rho*Vr^2*S_plate*Cl;
R_plate = sqrt(D_plate_vel^2 + L_plate^2);

% get the moment caused by the drag
% My_dp = l_plate*R_plate + l_plate*D_plate_rot;
Mz_dp = -(0.095+l_plate)*R_plate;
D_x = D_plate_vel*cos(heading);
D_y = D_plate_vel*sin(heading);

% get the forces caused by the drag
Fx_earth = -D_x;
Fy_earth = -D_y;
Fz_earth = -L_plate;

== matlab function B4_quadcopter_model_discrete/Discrete Model - Complementary Filtering/Force and Moment Calculation/Forces due to thrust ==
  data: omega_1 input; omega_2 input; F_t_e output; omega_3 input; omega_4 input; R_bg input; K_t input; F_t_b output
function [F_t_e,F_t_b] = F_t(omega_1, omega_2, omega_3, omega_4, R_bg, K_t)

f_1 = [0 0 -K_t * omega_1^2];
f_2 = [0 0 -K_t * omega_2^2]; 
f_3 = [0 0 -K_t * omega_3^2]; 
f_4 = [0 0 -K_t * omega_4^2];

F_t_e = R_bg * (f_1' + f_2' + f_3' + f_4');
F_t_b = (f_1(:,3) + f_2(:,3) + f_3(:,3) + f_4(:,3));

== matlab function B4_quadcopter_model_discrete/Discrete Model - Complementary Filtering/Force and Moment Calculation/Moments due to thrust ==
  data: omega input; omega_dot input; M_t output; G1 input; G2 input; sampling_time input; I input
function M_t = M_t(omega, omega_dot, G1, G2, sampling_time, I)

M_t = I * (0.5 * G1(1:3,:) * omega.^2 + sampling_time * G2 * omega_dot);

== matlab function B4_quadcopter_model_discrete/Discrete Model - Complementary Filtering/Plant and State Estimation/Plant Dynamics Continuous/body_to_ground_transorm ==
  data: Phi input; R_bg output; Theta input; Psi input
function R_bg  = R_bg(Phi,Theta,Psi)

% conventional rotation body to ground [312] or ZXY
% R_bg_312 = R_theta * R_phi * R_psi;
R_bg = [cos(Psi)*cos(Theta) cos(Psi)*sin(Phi)*sin(Theta) - cos(Phi)*sin(Psi) sin(Phi)*sin(Psi) + cos(Phi)*cos(Psi)*sin(Theta);
cos(Theta)*sin(Psi) cos(Phi)*cos(Psi) + sin(Phi)*sin(Psi)*sin(Theta) cos(Phi)*sin(Psi)*sin(Theta) - cos(Psi)*sin(Phi);
-sin(Theta) cos(Theta)*sin(Phi) cos(Phi)*cos(Theta)];

== matlab function B4_quadcopter_model_discrete/Discrete Model - Complementary Filtering/Plant and State Estimation/Plant Dynamics Continuous/euler_rates_to_pqr ==
  data: Phi input; R output; Theta input
function R = euler_rates_to_pqr(Phi,Theta)
R = [1 0 -sin(Theta);
0 cos(Phi) cos(Theta)*sin(Phi);
0 -sin(Phi) cos(Phi)*cos(Theta)];

== matlab function B4_quadcopter_model_discrete/Discrete Model - Complementary Filtering/Plant and State Estimation/Plant Dynamics Continuous/pqr_to_euler_rates ==
  data: Phi input; T output; Theta input
function T = pqr_to_euler_rates(Phi,Theta)
T = [1 (sin(Phi)*sin(Theta))/cos(Theta) (cos(Phi)*sin(Theta))/cos(Theta);
0 cos(Phi) -sin(Phi);
0 sin(Phi)/cos(Theta) cos(Phi)/cos(Theta)];

== matlab function B4_quadcopter_model_discrete/Discrete Model - Complementary Filtering/Plant and State Estimation/Plant Dynamics Continuous/wrapper ==
  data: pis_e input; psie_w output
function psie_w = wrapper(pis_e)

if pis_e > pi
    psie_w = pis_e - 2*pi;
elseif pis_e <= -pi
    psie_w = pis_e + 2*pi;
else
    psie_w = pis_e;
end

== matlab function B4_quadcopter_model_discrete/Discrete Model - Complementary Filtering/Plant and State Estimation/body_to_ground_transorm ==
  data: Phi input; R_bg output; Theta input; Psi input
function R_bg  = R_bg(Phi,Theta,Psi)

% conventional rotation body to ground [312] or ZXY
% R_bg_312 = R_theta * R_phi * R_psi;
R_bg = [cos(Psi)*cos(Theta) cos(Psi)*sin(Phi)*sin(Theta) - cos(Phi)*sin(Psi) sin(Phi)*sin(Psi) + cos(Phi)*cos(Psi)*sin(Theta);
cos(Theta)*sin(Psi) cos(Phi)*cos(Psi) + sin(Phi)*sin(Psi)*sin(Theta) cos(Phi)*sin(Psi)*sin(Theta) - cos(Psi)*sin(Phi);
-sin(Theta) cos(Theta)*sin(Phi) cos(Phi)*cos(Theta)];

== matlab function B4_quadcopter_model_discrete/Discrete Model/Force and Moment Calculation/Forces due to thrust ==
  data: omega_1 input; omega_2 input; F_t_e output; omega_3 input; omega_4 input; R_bg input; K_t input; F_t_b output
function [F_t_e,F_t_b] = F_t(omega_1, omega_2, omega_3, omega_4, R_bg, K_t)

f_1 = [0 0 -K_t * omega_1^2];
f_2 = [0 0 -K_t * omega_2^2]; 
f_3 = [0 0 -K_t * omega_3^2]; 
f_4 = [0 0 -K_t * omega_4^2];

F_t_e = R_bg * (f_1' + f_2' + f_3' + f_4');
F_t_b = (f_1(:,3) + f_2(:,3) + f_3(:,3) + f_4(:,3));

== matlab function B4_quadcopter_model_discrete/Discrete Model - Complementary Filtering/Plant and State Estimation/euler_rates_to_pqr ==
  data: Phi input; R output; Theta input
function R = euler_rates_to_pqr(Phi,Theta)
R = [1 0 -sin(Theta);
0 cos(Phi) cos(Theta)*sin(Phi);
0 -sin(Phi) cos(Phi)*cos(Theta)];

== matlab function B4_quadcopter_model_discrete/Discrete Model - Complementary Filtering/Plant and State Estimation/pqr_to_euler_rates ==
  data: Phi input; T output; Theta input
function T = pqr_to_euler_rates(Phi,Theta)
T = [1 (sin(Phi)*sin(Theta))/cos(Theta) (cos(Phi)*sin(Theta))/cos(Theta);
0 cos(Phi) -sin(Phi);
0 sin(Phi)/cos(Theta) cos(Phi)/cos(Theta)];

== matlab function B4_quadcopter_model_discrete/Discrete Model - Complementary Filtering/Plant and State Estimation/wrapper ==
  data: pis_e input; psie_w output
function psie_w = wrapper(pis_e)

if pis_e > pi
    psie_w = pis_e - 2*pi;
elseif pis_e <= -pi
    psie_w = pis_e + 2*pi;
else
    psie_w = pis_e;
end

== matlab function B4_quadcopter_model_discrete/Discrete Model - Complementary Filtering/Plant and State Estimation/wrapper1 ==
  data: pis_e input; psie_w output
function psie_w = wrapper(pis_e)

if pis_e > pi
    psie_w = pis_e - 2*pi;
elseif pis_e <= -pi
    psie_w = pis_e + 2*pi;
else
    psie_w = pis_e;
end

== matlab function B4_quadcopter_model_discrete/Discrete Model - Complementary Filtering/Plant and State Estimation/Angular Velocity Model/Moments due to thrust ==
  data: omega input; omega_dot input; M_t output; G1 input; G2 input; sampling_time input; I input
function M_t = M_t(omega, omega_dot, G1, G2, sampling_time, I)

M_t = I * (0.5 * G1(1:3,:) * omega.^2 + sampling_time * G2 * omega_dot);

== matlab function B4_quadcopter_model_discrete/Discrete Model - Complementary Filtering/Plant and State Estimation/Subsystem1/Forces due to thrust ==
  data: omega_1 input; omega_2 input; F_t_e output; omega_3 input; omega_4 input; R_bg input; K_t input; F_t_b output
function [F_t_e,F_t_b] = F_t(omega_1, omega_2, omega_3, omega_4, R_bg, K_t)

f_1 = [0 0 -K_t * omega_1^2];
f_2 = [0 0 -K_t * omega_2^2]; 
f_3 = [0 0 -K_t * omega_3^2]; 
f_4 = [0 0 -K_t * omega_4^2];

F_t_e = R_bg * (f_1' + f_2' + f_3' + f_4');
F_t_b = (f_1(:,3) + f_2(:,3) + f_3(:,3) + f_4(:,3));

== matlab function B4_quadcopter_model_discrete/Discrete Model/Discrete INDI Controller Cascaded w// Actuator Compensation/Subsystem/MATLAB Function ==
  data: theta input; qdd_comp output; dtheta input; Vx input; Vy input; Ax input; Ay input; w_plate input; h_plate input; l_plate input; Iyy input
function qdd_comp = fcn(theta,dtheta,Vx,Vy,Ax,Ay,w_plate,h_plate,l_plate,Iyy)

S_plate = w_plate * h_plate;
rho = 1.225;

% Cd = + 0.7 (correct)
qdd_comp = (Ax*l_plate*(S_plate^2*Vx*rho^2*(Vx^2 + Vy^2)*((513*theta)/(125*pi) + 21/500)^2 + S_plate^2*Vx*rho^2*(Vx^2 + Vy^2)*((297*theta)/(500*pi) + 997/1000)^2))/(2*Iyy*((S_plate^2*rho^2*(Vx^2 + Vy^2)^2*((513*theta)/(125*pi) + 21/500)^2)/4 + (S_plate^2*rho^2*(Vx^2 + Vy^2)^2*((297*theta)/(500*pi) + 997/1000)^2)/4)^(1/2)) + (Ay*l_plate*(S_plate^2*Vy*rho^2*(Vx^2 + Vy^2)*((513*theta)/(125*pi) + 21/500)^2 + S_plate^2*Vy*rho^2*(Vx^2 + Vy^2)*((297*theta)/(500*pi) + 997/1000)^2))/(2*Iyy*((S_plate^2*rho^2*(Vx^2 + Vy^2)^2*((513*theta)/(125*pi) + 21/500)^2)/4 + (S_plate^2*rho^2*(Vx^2 + Vy^2)^2*((297*theta)/(500*pi) + 997/1000)^2)/4)^(1/2)) + (dtheta*l_plate*((513*S_plate^2*rho^2*(Vx^2 + Vy^2)^2*((513*theta)/(125*pi) + 21/500))/(250*pi) + (297*S_plate^2*rho^2*(Vx^2 + Vy^2)^2*((297*theta)/(500*pi) + 997/1000))/(1000*pi)))/(2*Iyy*((S_plate^2*rho^2*(Vx^2 + Vy^2)^2*((513*theta)/(125*pi) + 21/500)^2)/4 + (S_plate^2*rho^2*(Vx^2 + Vy^2)^2*((297*theta)/(500*pi) + 997/1000)^2)/4)^(1/2));

== matlab function B4_quadcopter_model_discrete/Discrete Model - Complementary Filtering/Discrete INDI Controller Cascaded w// Actuator Compensation/Subsystem/MATLAB Function ==
  data: theta input; qdd_comp output; dtheta input; Vx input; Vy input; Ax input; Ay input; w_plate input; h_plate input; l_plate input; Iyy input
function qdd_comp = fcn(theta,dtheta,Vx,Vy,Ax,Ay,w_plate,h_plate,l_plate,Iyy)

S_plate = w_plate * h_plate;
rho = 1.225;

% Cd = + 0.7 (correct)
qdd_comp = (Ax*l_plate*(S_plate^2*Vx*rho^2*(Vx^2 + Vy^2)*((513*theta)/(125*pi) + 21/500)^2 + S_plate^2*Vx*rho^2*(Vx^2 + Vy^2)*((297*theta)/(500*pi) + 997/1000)^2))/(2*Iyy*((S_plate^2*rho^2*(Vx^2 + Vy^2)^2*((513*theta)/(125*pi) + 21/500)^2)/4 + (S_plate^2*rho^2*(Vx^2 + Vy^2)^2*((297*theta)/(500*pi) + 997/1000)^2)/4)^(1/2)) + (Ay*l_plate*(S_plate^2*Vy*rho^2*(Vx^2 + Vy^2)*((513*theta)/(125*pi) + 21/500)^2 + S_plate^2*Vy*rho^2*(Vx^2 + Vy^2)*((297*theta)/(500*pi) + 997/1000)^2))/(2*Iyy*((S_plate^2*rho^2*(Vx^2 + Vy^2)^2*((513*theta)/(125*pi) + 21/500)^2)/4 + (S_plate^2*rho^2*(Vx^2 + Vy^2)^2*((297*theta)/(500*pi) + 997/1000)^2)/4)^(1/2)) + (dtheta*l_plate*((513*S_plate^2*rho^2*(Vx^2 + Vy^2)^2*((513*theta)/(125*pi) + 21/500))/(250*pi) + (297*S_plate^2*rho^2*(Vx^2 + Vy^2)^2*((297*theta)/(500*pi) + 997/1000))/(1000*pi)))/(2*Iyy*((S_plate^2*rho^2*(Vx^2 + Vy^2)^2*((513*theta)/(125*pi) + 21/500)^2)/4 + (S_plate^2*rho^2*(Vx^2 + Vy^2)^2*((297*theta)/(500*pi) + 997/1000)^2)/4)^(1/2));

== matlab function B4_quadcopter_model_discrete/Discrete Model - Complementary Filtering/Discrete INDI Controller Cascaded w// Actuator Compensation/Subsystem/MATLAB Function1 ==
  data: theta input; rdd_comp output; dtheta input; Vx input; Vy input; Ax input; Ay input; w_plate input; h_plate input; l_plate input; Izz input
function rdd_comp = fcn(theta,dtheta,Vx,Vy,Ax,Ay,w_plate,h_plate,l_plate,Izz)

S_plate = w_plate * h_plate;
rho = 1.225;

% Cd = + 0.7 (correct)
rdd_comp = - (dtheta*((513*S_plate^2*rho^2*(Vx^2 + Vy^2)^2*((513*theta)/(125*pi) + 21/500))/(250*pi) + (297*S_plate^2*rho^2*(Vx^2 + Vy^2)^2*((297*theta)/(500*pi) + 997/1000))/(1000*pi))*(l_plate + 19/200))/(2*Izz*((S_plate^2*rho^2*(Vx^2 + Vy^2)^2*((513*theta)/(125*pi) + 21/500)^2)/4 + (S_plate^2*rho^2*(Vx^2 + Vy^2)^2*((297*theta)/(500*pi) + 997/1000)^2)/4)^(1/2)) - (Ax*(l_plate + 19/200)*(S_plate^2*Vx*rho^2*(Vx^2 + Vy^2)*((513*theta)/(125*pi) + 21/500)^2 + S_plate^2*Vx*rho^2*(Vx^2 + Vy^2)*((297*theta)/(500*pi) + 997/1000)^2))/(2*Izz*((S_plate^2*rho^2*(Vx^2 + Vy^2)^2*((513*theta)/(125*pi) + 21/500)^2)/4 + (S_plate^2*rho^2*(Vx^2 + Vy^2)^2*((297*theta)/(500*pi) + 997/1000)^2)/4)^(1/2)) - (Ay*(l_plate + 19/200)*(S_plate^2*Vy*rho^2*(Vx^2 + Vy^2)*((513*theta)/(125*pi) + 21/500)^2 + S_plate^2*Vy*rho^2*(Vx^2 + Vy^2)*((297*theta)/(500*pi) + 997/1000)^2))/(2*Izz*((S_plate^2*rho^2*(Vx^2 + Vy^2)^2*((513*theta)/(125*pi) + 21/500)^2)/4 + (S_plate^2*rho^2*(Vx^2 + Vy^2)^2*((297*theta)/(500*pi) + 997/1000)^2)/4)^(1/2));

== matlab function B4_quadcopter_model_discrete/Discrete Model - Inner Loop Only/Discrete INDI Controller Cascaded/ERROR CONTROLLER ATTITUDE/MATLAB Function1 ==
  data: pis_e input; psie_w output
function psie_w = wrapper(pis_e)

if pis_e > pi
    psie_w = pis_e - 2*pi;
elseif pis_e <= -pi
    psie_w = pis_e + 2*pi;
else
    psie_w = pis_e;
end

== matlab function B4_quadcopter_model_discrete/Discrete Model - Doublet/Discrete INDI Controller Cascaded/ERROR CONTROLLER ATTITUDE/MATLAB Function1 ==
  data: pis_e input; psie_w output
function psie_w = wrapper(pis_e)

if pis_e > pi
    psie_w = pis_e - 2*pi;
elseif pis_e <= -pi
    psie_w = pis_e + 2*pi;
else
    psie_w = pis_e;
end

== matlab function B4_quadcopter_model_discrete/Discrete Model - Doublet/Discrete INDI Controller Cascaded/G1+G2 ==
  data: G1 input; B_inner output; G2 input; omega input
function B_inner = B_inner(G1,G2,omega)

% add additional row to G2 for equal size
G2_T = [0 0 0 0];
G2 = vertcat(G2,G2_T);

B_inner = (G1 .* omega' + G2);

== matlab function B4_quadcopter_model_discrete/Discrete Model - Complementary Filtering/Discrete INDI Controller Cascaded/ERROR CONTROLLER ATTITUDE/MATLAB Function1 ==
  data: pis_e input; psie_w output
function psie_w = wrapper(pis_e)

if pis_e > pi
    psie_w = pis_e - 2*pi;
elseif pis_e <= -pi
    psie_w = pis_e + 2*pi;
else
    psie_w = pis_e;
end

== matlab function B4_quadcopter_model_discrete/Discrete Model - Doublet/Discrete INDI Controller Cascaded/G2_comp ==
  data: G2 input; domega input; G2_comp output
function G2_comp = G2_comp(G2,domega)

G2_comp = G2(3,:) * domega;

== matlab function B4_quadcopter_model_discrete/Discrete Model - Doublet/Discrete INDI Controller Cascaded/INTERNAL REFERENCE MODEL ATTITUDE/MATLAB Function1 ==
  data: pis_e input; psie_w output
function psie_w = wrapper(pis_e)

if pis_e > pi
    psie_w = pis_e - 2*pi;
elseif pis_e <= -pi
    psie_w = pis_e + 2*pi;
else
    psie_w = pis_e;
end

== matlab function B4_quadcopter_model_discrete/Discrete Model - Doublet/Discrete INDI Controller Cascaded/MATLAB Function1 ==
  data: T input; B_outer output; Phi input; Theta input; Psi input; m input
function B_outer = control_allocation_simple_outer(T,Phi,Theta,Psi,m)

B_outer = zeros(3,3);

% matrix obtained in ZXY rotation
% output order u = [phi theta thrust]
B_outer(1,1) = (T*cos(Phi)*cos(Psi)*cos(Theta))/m;
B_outer(2,1) = (T*cos(Phi)*cos(Theta)*sin(Psi))/m;
B_outer(3,1) = -(T*cos(Phi)*sin(Theta))/m;

B_outer(1,2) = (T*(cos(Phi)*sin(Psi) - cos(Psi)*sin(Phi)*sin(Theta)))/m;
B_outer(2,2) = -(T*(cos(Phi)*cos(Psi) + sin(Phi)*sin(Psi)*sin(Theta)))/m;
B_outer(3,2) = -(T*cos(Theta)*sin(Phi))/m;

B_outer(1,3) = (sin(Phi)*sin(Psi) + cos(Phi)*cos(Psi)*sin(Theta))/m;
B_outer(2,3) = -(cos(Psi)*sin(Phi) - cos(Phi)*sin(Psi)*sin(Theta))/m;
B_outer(3,3) = (cos(Phi)*cos(Theta))/m;

end

== matlab function B4_quadcopter_model_discrete/Discrete Model - Inner Loop Only/Discrete INDI Controller Cascaded/G1+G2 ==
  data: G1 input; B_inner output; G2 input
function B_inner = B_inner(G1,G2)

B_inner = (G1(1:3,:)+ G2);

== matlab function B4_quadcopter_model_discrete/Discrete Model - Doublet/Discrete INDI Controller Cascaded w// Actuator Compensation/ERROR CONTROLLER ATTITUDE/MATLAB Function1 ==
  data: pis_e input; psie_w output
function psie_w = wrapper(pis_e)

if pis_e > pi
    psie_w = pis_e - 2*pi;
elseif pis_e <= -pi
    psie_w = pis_e + 2*pi;
else
    psie_w = pis_e;
end

== matlab function B4_quadcopter_model_discrete/Discrete Model - Doublet/Discrete INDI Controller Cascaded w// Actuator Compensation/G1+G2 ==
  data: G1 input; B_inner output; G2 input; omega input; K_act input
function B_inner = B_inner(G1,G2,omega,K_act)

% add additional row to G2 for equal size
G2_T = [0 0 0 0];
G2 = vertcat(G2,G2_T);

B_inner = K_act*(G1 .* omega' + G2);

== matlab function B4_quadcopter_model_discrete/Discrete Model - Doublet/Discrete INDI Controller Cascaded w// Actuator Compensation/G2_comp ==
  data: G2 input; K_act input; domega input; G2_comp output
function G2_comp = G2_comp(G2,K_act,domega)

G2_comp = K_act * G2(3,:) * domega;

== matlab function B4_quadcopter_model_discrete/Discrete Model - Doublet/Discrete INDI Controller Cascaded w// Actuator Compensation/INTERNAL REFERENCE MODEL ATTITUDE/MATLAB Function1 ==
  data: pis_e input; psie_w output
function psie_w = wrapper(pis_e)

if pis_e > pi
    psie_w = pis_e - 2*pi;
elseif pis_e <= -pi
    psie_w = pis_e + 2*pi;
else
    psie_w = pis_e;
end

== matlab function B4_quadcopter_model_discrete/Discrete Model - Doublet/Discrete INDI Controller Cascaded w// Actuator Compensation/MATLAB Function1 ==
  data: T input; B_outer output; Phi input; Theta input; Psi input; m input
function B_outer = control_allocation_simple_outer(T,Phi,Theta,Psi,m)

B_outer = zeros(3,3);

% matrix obtained in ZXY rotation
% output order u = [phi theta thrust]
B_outer(1,1) = (T*cos(Phi)*cos(Psi)*cos(Theta))/m;
B_outer(2,1) = (T*cos(Phi)*cos(Theta)*sin(Psi))/m;
B_outer(3,1) = -(T*cos(Phi)*sin(Theta))/m;

B_outer(1,2) = (T*(cos(Phi)*sin(Psi) - cos(Psi)*sin(Phi)*sin(Theta)))/m;
B_outer(2,2) = -(T*(cos(Phi)*cos(Psi) + sin(Phi)*sin(Psi)*sin(Theta)))/m;
B_outer(3,2) = -(T*cos(Theta)*sin(Phi))/m;

B_outer(1,3) = (sin(Phi)*sin(Psi) + cos(Phi)*cos(Psi)*sin(Theta))/m;
B_outer(2,3) = -(cos(Psi)*sin(Phi) - cos(Phi)*sin(Psi)*sin(Theta))/m;
B_outer(3,3) = (cos(Phi)*cos(Theta))/m;

end
